simulink model "lab6_sec_5__PID"  (R2018a)
settings: Solver=VariableStepAuto  StartTime=0.0  StopTime=10  MaxStep=0.001  RelTol=1e-3
libraries: ECEN315_Library x2, powerlib x2, ECEN315_Library_Fault x1
settings Model: Creator=joshua  LastModifiedBy=joshua

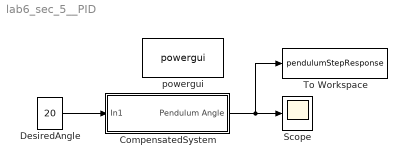
== system lab6_sec_5__PID ==
  CompensatedSystem : Subsystem  mask{Kp=0.505, Ki=0, Kd=0.3}
  DesiredAngle : Constant  Value=20  VectorParams1D=off  OutDataTypeStr=double
  Scope : Scope
  To Workspace : ToWorkspace  VariableName=pendulumStepResponse  SampleTime=-1
      settings: Save2DSignal=2-D array (concatenate along first dimension)
  powergui : powerlib/powergui  Priority=1  SimulationMode=Continuous  SampleTime=50e-6  frequency=60  Iterations=50  frequencyindice=0  Pbase=100e6  ErrMax=1e-4  UnitsV=kV  UnitsW=MW  buscounter=0  FunctionMessages=off  echomessages=off  EnableUseOfTLC=off  CurrentSourceSwitches=off  DisableSnubberDevices=off  DisableRonSwitches=off  DisableVfSwitches=off  DisplayEquations=off  SolverType=Tustin/Backward Euler (TBE)  Interpol=off  ExternalGateDelay=off  methode=off  Ts=100  x0status=blocks  SPID=on  SwTol=0  HookPort=off  RestoreLinks=warning  ResistiveCurrentMeasurement=off  Frange=[0:2:500]  Ylog=off  Xlog=on  ShowGrid=off  save=off  variable=ZData  structure=0  ZoomFFT=off  StartTime=0.0  cycles=1  DisplayStyle=1  fundamental=60  FreqAxis=off  MaxFrequency=1000  frequencyindicesteady=1  RmsSteady=1  display=off
  wires:
  CompensatedSystem/1(Pendulum Angle) -> To Workspace/1, Scope/1
  DesiredAngle/1 -> CompensatedSystem/1(In1)

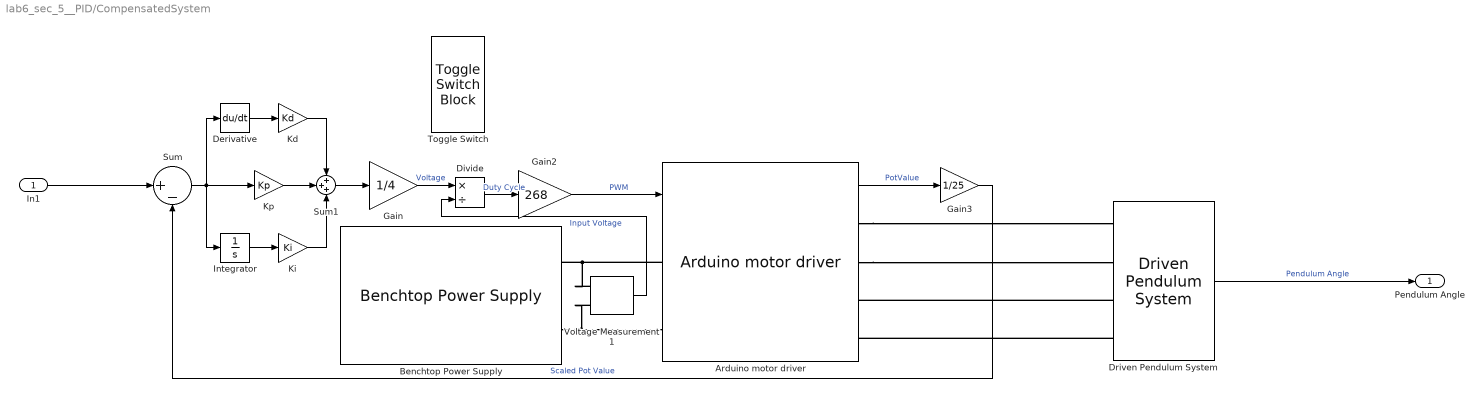
== system lab6_sec_5__PID/CompensatedSystem ==
  In1 : Inport
  Arduino motor driver : ECEN315_Library_Fault/Arduino motor driver  E=off
  Benchtop Power Supply : ECEN315_Library/Benchtop Power Supply  V=12
  Derivative : Derivative
  Divide : Product  Inputs=*/
  Driven Pendulum System : ECEN315_Library/Driven Pendulum System  SystemSampleTime=-1
  Gain : Gain  Gain=1/4
  Gain2 : Gain  Gain=268
  Gain3 : Gain  Gain=1/25
  Integrator : Integrator
  "Kd " : Gain  Gain=Kd
  "Ki " : Gain  Gain=Ki
  "Kp " : Gain  Gain=Kp
  Sum : Sum  Inputs=|+-
  Sum1 : Sum  Inputs=+++
  Toggle Switch : ToggleSwitchBlock  WebBlockId=55
      settings: Values={{'Off', 'On'}, [0 12]}
  Voltage Measurement1 : powerlib/Measurements/Voltage Measurement  PhasorSimulation=off  OutputType=Complex  PSBequivalent=0
  Pendulum Angle : Outport
  wires:
  Gain/1 -> Divide/1  "Voltage"
  Derivative/1 -> "Kd "/1
  Integrator/1 -> "Ki "/1
  Divide/1 -> Gain2/1  "Duty Cycle"
  Arduino motor driver/1 -> Gain3/1  "PotValue"
  "Kp "/1 -> Sum1/2
  "Ki "/1 -> Sum1/3
  In1/1 -> Sum/1
  Driven Pendulum System/1 -> Pendulum Angle/1  "Pendulum Angle"
  Sum/1 -> Integrator/1, Derivative/1, "Kp "/1
  Sum1/1 -> Gain/1
  "Kd "/1 -> Sum1/1
  Voltage Measurement1/1 -> Divide/2  "Input Voltage"
  Gain2/1 -> Arduino motor driver/1  "PWM"
  Gain3/1 -> Sum/2  "Scaled Pot Value"
  connections:
  Benchtop Power Supply/RConn2 -- Voltage Measurement1/LConn2 -- Arduino motor driver/LConn2
  Arduino motor driver/LConn1 -- Voltage Measurement1/LConn1 -- Benchtop Power Supply/RConn1
  Arduino motor driver/RConn1 -- Driven Pendulum System/LConn1
  Arduino motor driver/RConn2 -- Driven Pendulum System/LConn2
  Driven Pendulum System/LConn4 -- Arduino motor driver/RConn4
  Driven Pendulum System/LConn3 -- Arduino motor driver/RConn3
